simulink model "data_recording"  (R2024a)
settings: Solver=FixedStepAuto  StartTime=0.0  StopTime=120  FixedStep=Ts  RelTol=1e-3  EnableMultiTasking=on
libraries: raspberrypiCommlib x2, statsLibrary x1, dspfdesign x1
settings Model: SimulationMode=external  ExtModeTrigDuration=2  Creator=Benutzer  LastModifiedBy=s2310825007
settings SolverCC: PositivePriorityOrder=on
settings DataIOCC: ReturnWorkspaceOutputs=off
settings OptimizationCC: EnhancedBackFolding=on  PassReuseOutputArgsAs=Individual arguments  ZeroExternalMemoryAtStartup=off  ZeroInternalMemoryAtStartup=off  MaxStackSize=64  DifferentSizesBufferReuse=on  EfficientTunableParamExpr=on
settings DebuggingCC: ParameterTunabilityLossMsg=error
settings HardwareCC: ProdBitPerPointer=32  ProdBitPerSizeT=32  ProdBitPerPtrDiffT=32  ProdLargestAtomicInteger=Long  ProdLargestAtomicFloat=Double  ProdWordSize=32  ProdLongLongMode=on  ProdHWDeviceType=ARM Compatible->ARM Cortex
settings RTWCC: Description=Embedded Coder  SystemTargetFile=ert.tlc  HardwareBoard=Raspberry Pi  TemplateMakefile=ert_default_tmf  Toolchain=GNU GCC Embedded Linux  BuildConfiguration=Faster Runs  GPUComputeCapability=3.5
settings CodeAppCC: ForceParamTrailComments=on  IgnoreCustomStorageClasses=off  OperatorAnnotations=on  SimulinkDataObjDesc=on  SFDataObjDesc=on  InsertBlockDesc=on
settings ERTTargetCC: SupportVariableSizeSignals=on  ExtMode=on  ExtModeTransport=2  ExtModeStaticAlloc=on  ExtModeMaxTrigDuration=1000  ExtModeMexFile=ext_xcp  ExtModeMexArgs='CM7' 0 17725  ExtModeIntrfLevel=Level2 - Open

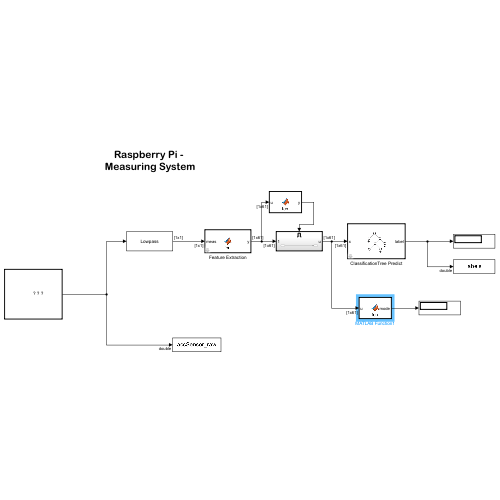
[thumbnail: Simulink's stored preview of the top-level diagram]
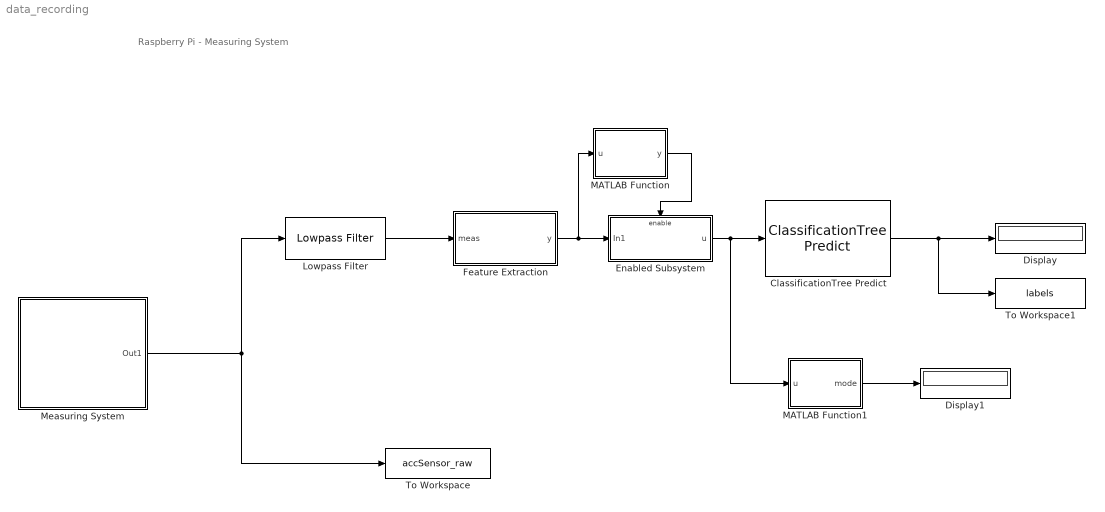
== system data_recording ==
  note: Raspberry Pi -
      | Measuring System
  ClassificationTree Predict : statsLibrary/Classification/ClassificationTree Predict  TrainedLearner=trainedModel5.ClassificationTree  ShowOutputScore=off  LabelDataTypeStr=Inherit: Inherit via back propagation  LabelOutMin=[]  LabelOutMax=[]  ScoreOutMin=[]  ScoreOutMax=[]  RawScoreOutMin=[]  RawScoreOutMax=[]  StoredEnumName=treeMdl_enumLabels
  Display : Display
  Display1 : Display
  Enabled Subsystem : Subsystem  TreatAsAtomicUnit=on
  Feature Extraction : MATLAB Function  TreatAsAtomicUnit=on  mask{StreamingFunction=diagnosticFeatures4, BufferSize=10001, BufferOverlap=0, SigIV=Time, StartTime=0, SamplingRate=1e3, IVSignal=IVSignal, InputNames=meas, NumFeatures=61}
      mask prompts: StreamingFunction "predmaint:plot:maskParamFuncName"; BufferSize "predmaint:plot:maskParamBufferSize"; BufferOverlap "predmaint:plot:maskParamBufferOverlap"; SigIV "predmaint:plot:dlgIVTypeLabel"; StartTime "predmaint:plot:maskParamStartTime"; SamplingRate "predmaint:plot:maskParamSamplingRate"; IVSignal "predmaint:plot:maskParamSignalName"; InputNames "predmaint:plot:maskInputNames"; NumFeatures "predmaint:plot:maskNumOfFeatures"
      mask help:
      | Imitates the feature extraction process performed in the Diagnostic Feature Designer (DFD) app. Only computes a set of top features that the block was created to extract and provides the result as a vector output.
      |
      | Streaming Function Name: The name of the function that will be used for feature computation.
      |
      | Buffer Size: The size of the signals/spectra on which feature computation will be performed.
      |
      | Buffer Overlap: The size of the signals/spectra that will be re-used for consecutive feature computation.
      |
      | IV Type: Select an Independent Variable for feature computation. It can be either Time (with its own Start Time and Sampling Rate) or an additional Signal input to the block.
      mask init:
      | predmaintguis.internal.ciapp.dialogs.GenerateFeatureExtractionSimulinkBlock.cbInitialization(gcb);
  Lowpass Filter : dspfdesign/Lowpass Filter  FilterType=FIR  DesignForMinimumOrder=on  FilterOrder=50  PassbandFrequency=0.1  StopbandFrequency=200  PassbandRipple=0.1  StopbandAttenuation=80  SampleRateMode=Specify on dialog  SampleRate=1e3  SimulateUsing=Interpreted execution  roundingMode=Floor  coeffsDataTypeStr=fixdt(1,16)
  MATLAB Function : MATLAB Function  TreatAsAtomicUnit=on
  MATLAB Function1 : MATLAB Function  TreatAsAtomicUnit=on
  Measuring System : Subsystem
      mask Display: image('MeasuringSystem.PNG'); % Use "Edit Image" on toolstrip to change.
  To Workspace : ToWorkspace  VariableName=accSensor_raw  SaveFormat=Structure With Time  SampleTime=-1
      settings: Save2DSignal=2-D array (concatenate along first dimension)
  To Workspace1 : ToWorkspace  VariableName=labels  SaveFormat=Structure With Time  SampleTime=-1
  wires:
  ClassificationTree Predict/1 -> To Workspace1/1, Display/1
  Measuring System/1(Out1) -> Lowpass Filter/1, To Workspace/1
  Lowpass Filter/1 -> Feature Extraction/1(meas)
  Feature Extraction/1(y) -> MATLAB Function/1(u), Enabled Subsystem/1(In1)
  Enabled Subsystem/1(u) -> MATLAB Function1/1(u), ClassificationTree Predict/1
  MATLAB Function/1(y) -> Enabled Subsystem/Enable
  MATLAB Function1/1(mode) -> Display1/1

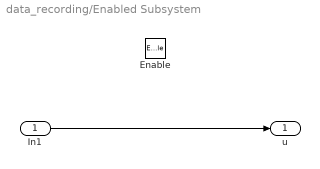
== system data_recording/Enabled Subsystem ==
  In1 : Inport
  Enable : EnablePort
  u : Outport
  wires:
  In1/1 -> u/1

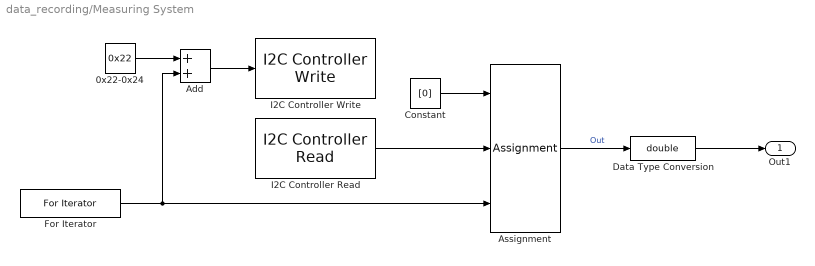
== system data_recording/Measuring System ==
  0x22-0x24 : Constant  Value=0x22  OutDataTypeStr=uint8  SampleTime=-1
  Add : Sum
  Assignment : Assignment  IndexMode=Zero-based  DiagnosticForDimensions=Warning  IndexOptions=Index vector (port)  Indices=1  OutputSizes=1
  Constant : Constant  Value=[0]  OutDataTypeStr=uint16  SampleTime=-1
  Data Type Conversion : DataTypeConversion  OutDataTypeStr=double  SaturateOnIntegerOverflow=off  RndMeth=Floor
  For Iterator : ForIterator  IterationLimit=1  IndexMode=Zero-based  IterationVariableDataType=uint8
  I2C Controller Read : raspberrypiCommlib/I2C Controller Read  BoardProperty=Pi 4 Model B  I2CModule=1  Mode=Master  SlaveAddress=8  SlaveByteOrder=LittleEndian  Direction=Receiver  RegisterAddressMode=off  RegisterAddress=uint8(0x22)  SlaveDataType=uint16  DataLength=1  NoAck=off  RepeatedStart=off  OutputStatus=off  SampleTime=-1
  I2C Controller Write : raspberrypiCommlib/I2C Controller Write  BoardProperty=Pi 4 Model B  I2CModule=1  Mode=Master  SlaveAddress=8  SlaveByteOrder=LittleEndian  Direction=Transmitter  RegisterAddressMode=off  RegisterAddress=0  SlaveDataType=uint8  DataLength=1  NoAck=off  RepeatedStart=off  OutputStatus=off
  Out1 : Outport
  wires:
  I2C Controller Read/1 -> Assignment/2
  For Iterator/1 -> Assignment/3, Add/2
  Constant/1 -> Assignment/1
  Add/1 -> I2C Controller Write/1
  0x22-0x24/1 -> Add/1
  Assignment/1 -> Data Type Conversion/1  "Out"
  Data Type Conversion/1 -> Out1/1

== matlab function data_recording/Feature Extraction ==
  data: meas input; y output
function y = fcn(meas)
persistent BufferData;
if isempty(BufferData)
BufferData = zeros(0,nargin);
end
BufferData = [BufferData;[meas]];
y = zeros(1,61);
BufferSize = 10001;
BufferOverlap = 0;
if size(BufferData,1) == BufferSize
StartTime = 0;
SamplingRate = 1e3;
EndTime = (SamplingRate*BufferSize+StartTime-SamplingRate);
meas = BufferData(:,1);
InputData = timetable(seconds(StartTime:SamplingRate:EndTime)',meas,'VariableNames',{'meas'});
tbl = diagnosticFeatures4(InputData);
y = table2array(tbl);
if size(BufferData,2)>1 
BufferData(1:(BufferSize-BufferOverlap),:) = [];
else 
BufferData(1:(BufferSize-BufferOverlap)) = [];
end
end
end

== matlab function data_recording/MATLAB Function1 ==
  data: u input; mode output
function mode = fcn(u)
    classifier = loadLearnerForCoder("trainedModel5.mat");
    mode = predict(classifier, u);

== matlab function data_recording/MATLAB Function ==
  data: u input; y output
function y = fcn(u)
    y = u(1)~=0 & u(2)~=0;
